simulink model "satellite8"  (Simulink 7.5)
settings: Solver=ode45  StartTime=0.0  StopTime=10.0  RelTol=1e-3
libraries: simulink_extras x3, dspswit3 x3, commsynccomp2 x2, commchan3 x1, dspsrcs4 x1
settings Model: Creator=sisa  LastModifiedBy=sisa

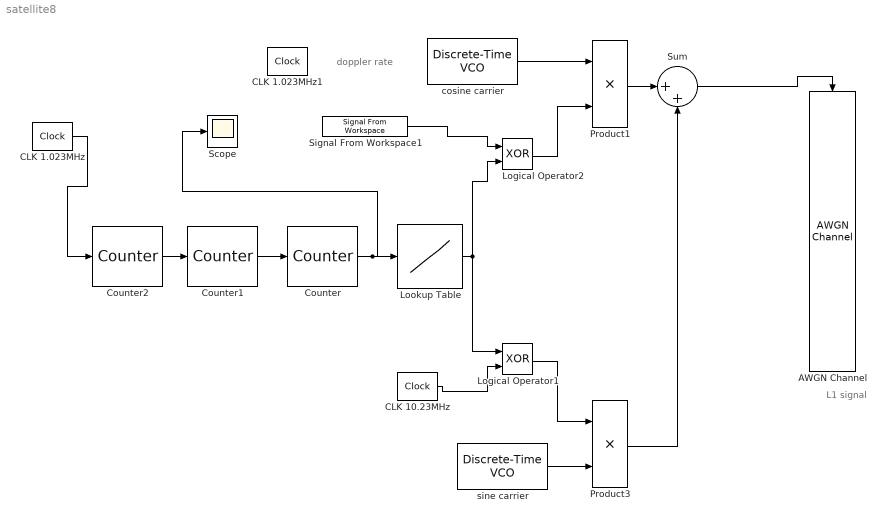
== system satellite8 ==
  note: doppler rate
  note: L1 signal
  AWGN Channel : commchan3/AWGN Channel  SystemSampleTime=-1  seed=67  noiseMode="Signal to noise ratio  (Eb/No)"  EbNodB=10  EsNodB=10  SNRdB=10  bitsPerSym=1  Ps=1  Tsym=1  variance=1
  CLK 1.023MHz : simulink_extras/Flip Flops/Clock  SystemSampleTime=-1  MaskParam1=9.7751e-7
  CLK 1.023MHz1 : simulink_extras/Flip Flops/Clock  SystemSampleTime=-1  MaskParam1=9.7751e-7
  CLK 10.23MHz : simulink_extras/Flip Flops/Clock  SystemSampleTime=-1  MaskParam1=0.00000009775
  Counter : dspswit3/Counter  Direction=Up  CountEvent=Rising edge  CounterSize=User defined  MaxCount=1500  InitialCount=0  Output=Count  HitValue=32  ResetInput=off  SamplesPerFrame=1  Ts=1  CntDtype=double  HitDtype=Logical
  Counter1 : dspswit3/Counter  Direction=Up  CountEvent=Rising edge  CounterSize=User defined  MaxCount=20  InitialCount=0  Output=Count  HitValue=32  ResetInput=off  SamplesPerFrame=1  Ts=1  CntDtype=double  HitDtype=Logical
  Counter2 : dspswit3/Counter  Direction=Up  CountEvent=Falling edge  CounterSize=User defined  MaxCount=1022  InitialCount=0  Output=Count  HitValue=32  ResetInput=off  SamplesPerFrame=1  Ts=1  CntDtype=double  HitDtype=Logical
  Logical Operator1 : Logic  Operator=XOR  AllPortsSameDT=off  OutDataTypeMode=boolean  LogicDataType=fixdt(0, 8)  OutDataTypeStr=boolean
  Logical Operator2 : Logic  Operator=XOR  AllPortsSameDT=off  OutDataTypeMode=boolean  LogicDataType=fixdt(0, 8)  OutDataTypeStr=boolean
  Lookup Table : Lookup  InputValues=[-5:5]  Table=tanh([-5:5])  LookUpMeth=Use Input Below  OutDataType=fixdt(1, 16)  OutScaling=2^0
  Product1 : Product  OutDataType=fixdt(1, 16)  OutScaling=2^0  RndMeth=Zero
  Product3 : Product  OutDataType=fixdt(1, 16)  OutScaling=2^0  RndMeth=Zero
  Scope : Scope
      settings: TimeRange=10  YMin=16  YMax=16
  Signal From Workspace1 : dspsrcs4/Signal From Workspace  SystemSampleTime=-1  X=PN08  Ts=1  nsamps=1  OutputAfterFinalValue=Setting to zero  ignoreOrWarnInputAndFrameLengths=off
  Sum : Sum  Inputs=|++  OutDataType=fixdt(1, 16)  OutScaling=2^0
  cosine carrier : commsynccomp2/Discrete-Time VCO  SystemSampleTime=-1  Ac=1  Fc=10e6  Kc=1  Ph=0  ts=0.01
  sine carrier : commsynccomp2/Discrete-Time VCO  SystemSampleTime=-1  Ac=1  Fc=10e6  Kc=1  Ph=0  ts=0.01
  wires:
  Logical Operator2/1 -> Product1/2
  Lookup Table/1 -> Logical Operator2/2, Logical Operator1/1
  Logical Operator1/1 -> Product3/1
  CLK 1.023MHz/1 -> Counter2/1
  Counter2/1 -> Counter1/1
  Counter1/1 -> Counter/1
  Counter/1 -> Lookup Table/1, Scope/1
  Signal From Workspace1/1 -> Logical Operator2/1
  sine carrier/1 -> Product3/2
  cosine carrier/1 -> Product1/1
  ? -> cosine carrier/1, sine carrier/1
  CLK 10.23MHz/1 -> Logical Operator1/2
  Product3/1 -> Sum/2
  Product1/1 -> Sum/1
  Sum/1 -> AWGN Channel/1
